simulink library "CAU_NXP_Car_Lib"  (R2016a)
settings: Solver=ode45  StartTime=0.0  StopTime=10.0  RelTol=1e-3
undefined symbols (not defined in the file or in its folder): s
settings Model: Creator=tfuser  LastModifiedBy=tfuser
settings DataIOCC: LimitDataPoints=on  SaveFormat=Array
settings DebuggingCC: AllowSymbolicDim=off
settings HardwareCC: ProdBitPerPointer=32  ProdLargestAtomicFloat=None  ProdIntDivRoundTo=Undefined  ProdEndianess=Unspecified  ProdWordSize=32  ProdHWDeviceType=32-bit Generic
settings ModelReferenceCC: PropagateSignalLabelsOutOfModel=off
settings ConfigComp: CovModelRefEnable=Off

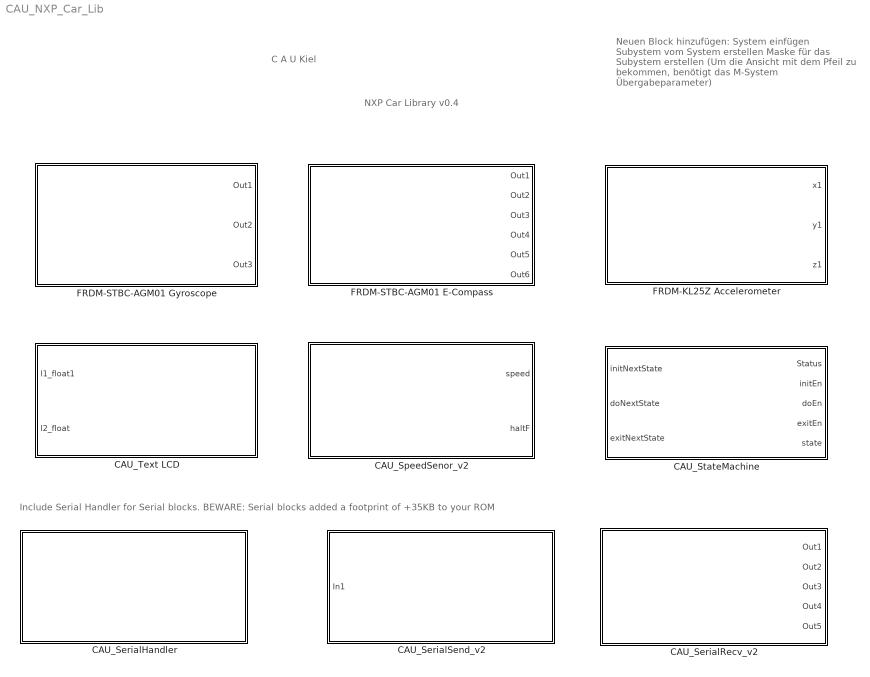
== system CAU_NXP_Car_Lib ==
  note: Include Serial Handler for Serial blocks. BEWARE: Serial blocks added a footprint of +35KB to your ROM
  note: Neuen Block hinzufügen:
      | System einfügen
      | Subystem vom System erstellen
      | Maske für das Subystem erstellen
      | (Um die Ansicht mit dem Pfeil zu bekommen,
      | benötigt das M-System Übergabeparameter)
  note: NXP Car Library v0.4
  note: C A U Kiel
  CAU_SerialHandler : Subsystem  mask{switchUART=0}
      mask prompts: switchUART "Switch UART (not implemented!)"
      mask help:
      | CAU_SerialHandler
      | Provides the pointer management to avoid two instances of mbeds serial object.
      mask TypeOptions switchUART: MATLAB System/switchUART
      mask Display:
      | pic = imread('resources/CAU_SerialHandler.png');
      | image(pic);
  CAU_SerialRecv_v2 : Subsystem  mask{quantToRecv=2, fullDigits=3, deciDigits=2, SampleTime=0.1}
      mask prompts: quantToRecv "Quantity of expected floating point numbers:"; fullDigits "Full Digits:"; deciDigits "Fractional digits:"; SampleTime "Simulink:blkprm_prompts:AllSrcBlksSampleTime"
      mask help:
      | Recieves serial data over UART/BT interface. The expected quantity parameter is crucial to match the incomming number of floats to act non-blocking! Output size is hard coded to 5* and output will be zero if there are less incomming numbers.
      |
      | Expected message format (ASCII coding): >+XXX.xx -YYY.yy ...
      | (Start char: ">", Seperator: Whitespace)
      |
      | * this output size is hard coded as constant property, as dealing with dynamic output length is not well supported by Simulink Coder.
      mask TypeOptions quantToRecv: MATLAB System/quantToRecv
      mask TypeOptions fullDigits: MATLAB System/fullDigits
      mask TypeOptions deciDigits: MATLAB System/deciDigits
      mask TypeOptions SampleTime: Constant1/SampleTime
      mask Display:
      | pic = imread('resources/SLBlock_Serial_Recv.png');
      | image(pic);
      | 
      | port_label('output',1,'f1');
      | port_label('output',2,'f2');
      | port_label('output',3,'f3');
      | port_label('output',4,'f4');
      | port_label('output',5,'f5');
  CAU_SerialSend_v2 : Subsystem  mask{quantToTrnf=2}
      mask prompts: quantToTrnf "Quantity to transfer:"
      mask help:
      | Sends a vector of floating points via UART/Bluetooth.
      | Numbers are formated to "+XXX.xx" with no range limitations (E-Notation is used)
      | Include State Machine!
      mask TypeOptions quantToTrnf: MATLAB System/quantToTrnf
      mask Display:
      | pic = imread('resources/SLBlock_Serial_Send.png');
      | image(pic);
      | 
      | port_label('input',1,'numVec');
  CAU_SpeedSenor_v2 : Subsystem  mask{WhichSensor=Left, SgmntWdth=36, ElpsdTMax=400, ChrTPT1=1/5, SampleTime=0.01}
      mask prompts: WhichSensor "Select Sensor:"; SgmntWdth "Segement width between two magnets in mm:"; ElpsdTMax "Maximum elapsed time in ms before stillstand detection, [300, 800]:"; ChrTPT1 "PT1 low pass: characteristic factor in respect to the block sample time [0, 10]:"; SampleTime "Simulink:blkprm_prompts:AllSrcBlksSampleTime"
      mask help: Measure car speed with magnets mounted inside the wheel.
      mask TypeOptions WhichSensor: MATLAB System/WhichSensor
      mask TypeOptions SgmntWdth: MATLAB System/SgmntWdth
      mask TypeOptions ElpsdTMax: MATLAB System/ElpsdTMax
      mask TypeOptions ChrTPT1: MATLAB System/ChrTPT1
      mask TypeOptions SampleTime: Constant1/SampleTime
      mask Display:
      | pic = imread('resources/speedsensor.png');
      | image(pic);
      | 
      | port_label('output',1,'speed');
      | port_label('output',2,'haltFlag');
  CAU_StateMachine : Subsystem  mask{SampleTime=0.1}
      mask prompts: SampleTime "Simulink:blkprm_prompts:AllSrcBlksSampleTime"
      mask TypeOptions SampleTime: Constant1/SampleTime
      mask Display:
      | pic = imread('resources/CAU_StateMachine.png');
      | image(pic);
      | 
      | port_label('output',1,'status');
      | port_label('output',2,'initEn');
      | port_label('output',3,'doEn');
      | port_label('output',4,'exitEn');
      | 
      | port_label('output',5,'state');
      | 
      | port_label('input',1,'initNext');
      | port_label('input',2,'doNext');
      | port_label('input',3,'exitNext');
  CAU_Text LCD : Subsystem  mask(Text LCD Display){}
      mask help:
      | TextLCD: print two floating numbers to the two lines of a HD44780 display
      |
      | IMPORTANT: add "-u_printf_float -u_scanf_float" to your <Linker> and <C++ Linker> options.
      |
      | Connected PINs : {PTC0}RS, {PTC7}E, {PTB8,PTB9,PTB10,PTB11}Data.
      | (TODO: To reduce the cables to two use a I2C implementation)
      mask Display:
      | pic = imread('resources/lcd.png');
      | image(pic);
      | 
      | port_label('input',1,'line1');
      | port_label('input',2,'line2');
  FRDM-KL25Z Accelerometer : Subsystem  SystemSampleTime=SystemSampleTime  mask(Accelerometer){WhichScale=+-2G, SystemSampleTime=-1, SampleTime=0.1}
      mask prompts: WhichScale "Full Scale:"; SystemSampleTime "Simulink:blkprm_prompts:AllBlksSampleTime"; SampleTime "Simulink:blkprm_prompts:AllSrcBlksSampleTime"
      mask help:
      | This Block reads out the data from the Accelerometer that is on the FRDM-KL25Z.
      |
      | Outputs 1-3 are the acceleration in x, y and z axis in m/(s^2).
      mask TypeOptions WhichScale: MATLAB System/WhichScale
      mask TypeOptions SystemSampleTime: SystemSampleTime
      mask TypeOptions SampleTime: CONST_g/SampleTime
      mask Display:
      | pic = imread('resources/acc_int.png');
      | image(pic);
      | 
      | port_label('output',1,'accel_x');
      | port_label('output',2,'accel_y');
      | port_label('output',3,'accel_z');
  FRDM-STBC-AGM01 E-Compass : Subsystem  SystemSampleTime=SystemSampleTime  mask(Accelerometer and Magnetometer){WhichScale=+-2G, SystemSampleTime=-1, SampleTime=0.1}
      mask prompts: WhichScale "Acc Full Scale:"; SystemSampleTime "Simulink:blkprm_prompts:AllBlksSampleTime"; SampleTime "Simulink:blkprm_prompts:AllSrcBlksSampleTime"
      mask help:
      | This Block reads out the data from the FXOS8700C 6-axis integrated e-compass that is on the FRDM-STBC-AGM01 Sensor Fusion Board.
      |
      | It reads out the values of the Accelerometer and the Magnetometer.
      | Outputs 1-3 are the acceleration in x, y and z axis in m/(s^2).
      | Outputs 4-6 are the magnetudes in x, y and z axis in uT.
      mask TypeOptions WhichScale: MATLAB System1/WhichScale
      mask TypeOptions SystemSampleTime: SystemSampleTime
      mask TypeOptions SampleTime: Constant1/SampleTime
      mask Display:
      | pic = imread('resources/acc_mag.png');
      | image(pic);
      | 
      | port_label('output',1,'accel_x');
      | port_label('output',2,'accel_y');
      | port_label('output',3,'accel_z');
      | port_label('output',4,'mag_x');
      | port_label('output',5,'mag_y');
      | port_label('output',6,'mag_z');
  FRDM-STBC-AGM01 Gyroscope : Subsystem  SystemSampleTime=SystemSampleTime  mask(Gyroscope){WhichScale=+-500rad/s, SystemSampleTime=-1, SampleTime=0.1}
      mask prompts: WhichScale "Full Scale:"; SystemSampleTime "Simulink:blkprm_prompts:AllBlksSampleTime"; SampleTime "Simulink:blkprm_prompts:AllSrcBlksSampleTime"
      mask help:
      | This Block reads out the data from the FXAS21002C 3-axis Gyroscope that is on the FRDM-STBC-AGM01 Sensor Fusion Board.
      |
      | It reads out the values of the Gyroscope.
      | Outputs 1-3 are the gyro-data in x, y and z axis in rad/s.
      mask TypeOptions WhichScale: MATLAB System/WhichScale
      mask TypeOptions SystemSampleTime: SystemSampleTime
      mask TypeOptions SampleTime: Constant1/SampleTime
      mask Display:
      | pic = imread('resources/gyro.png');
      | image(pic);
      | 
      | port_label('output',1,'gyro_x');
      | port_label('output',2,'gyro_y');
      | port_label('output',3,'gyro_z');

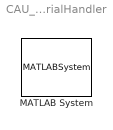
== system CAU_NXP_Car_Lib/CAU_SerialHandler ==
  MATLAB System : MATLABSystem  System=CAU_SerialHandler  switchUART=switchUART  SimulateUsing=Code generation
      mask Type: CAU_SerialHandler
      mask Display: disp('CAU_SerialHandler');

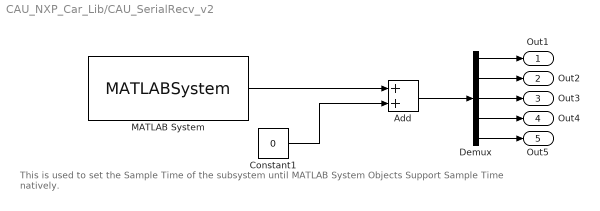
== system CAU_NXP_Car_Lib/CAU_SerialRecv_v2 ==
  note: This is used to set the Sample Time of the subsystem until MATLAB System Objects Support Sample Time natively.
  Add : Sum  AccumDataTypeStr=single
  Constant1 : Constant  Value=0  OutDataTypeStr=single  SampleTime=SampleTime
  Demux : Demux  Outputs=5
  MATLAB System : MATLABSystem  System=CAU_SerialRecv  quantToRecv=quantToRecv  fullDigits=fullDigits  deciDigits=deciDigits  SimulateUsing=Code generation
      mask Type: CAU_SerialRecv
      mask Display:
      | disp('CAU_SerialRecv');
      | port_label('output',1,'res');
  Out1 : Outport
  Out2 : Outport  Port=2
  Out3 : Outport  Port=3
  Out4 : Outport  Port=4
  Out5 : Outport  Port=5
  wires:
  Constant1/1 -> Add/2
  MATLAB System/1 -> Add/1
  Add/1 -> Demux/1
  Demux/1 -> Out1/1
  Demux/2 -> Out2/1
  Demux/3 -> Out3/1
  Demux/4 -> Out4/1
  Demux/5 -> Out5/1

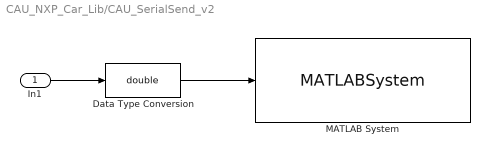
== system CAU_NXP_Car_Lib/CAU_SerialSend_v2 ==
  In1 : Inport
  Data Type Conversion : DataTypeConversion  OutDataTypeStr=double
  MATLAB System : MATLABSystem  System=CAU_SerialSend  quantToTrnf=quantToTrnf  SimulateUsing=Code generation
      mask Type: CAU_SerialSend
      mask Display:
      | disp('CAU_SerialSend');
      | port_label('input',1,'numVec');
  wires:
  In1/1 -> Data Type Conversion/1
  Data Type Conversion/1 -> MATLAB System/1

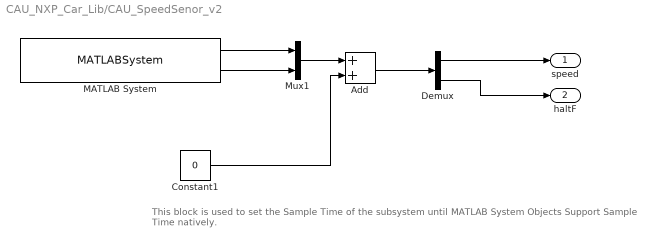
== system CAU_NXP_Car_Lib/CAU_SpeedSenor_v2 ==
  note: This block is used to set the Sample Time of the subsystem until MATLAB System Objects Support Sample Time natively.
  Add : Sum  AccumDataTypeStr=single
  Constant1 : Constant  Value=0  OutDataTypeStr=single  SampleTime=SampleTime
  Demux : Demux  Outputs=2
  MATLAB System : MATLABSystem  System=CAU_SpeedSensor  SgmntWdth=SgmntWdth  ElpsdTMax=ElpsdTMax  ChrTPT1=ChrTPT1  WhichSensor=Left  SimulateUsing=Code generation
      mask Type: CAU_SpeedSensor
      mask Display:
      | disp('CAU_SpeedSensor');
      | port_label('output',1,'speed');
      | port_label('output',2,'stillstand');
  Mux1 : Mux  Inputs=2
  speed : Outport
  haltF : Outport  Port=2
  wires:
  Constant1/1 -> Add/2
  Mux1/1 -> Add/1
  MATLAB System/2 -> Mux1/2
  Add/1 -> Demux/1
  Demux/2 -> haltF/1
  MATLAB System/1 -> Mux1/1
  Demux/1 -> speed/1

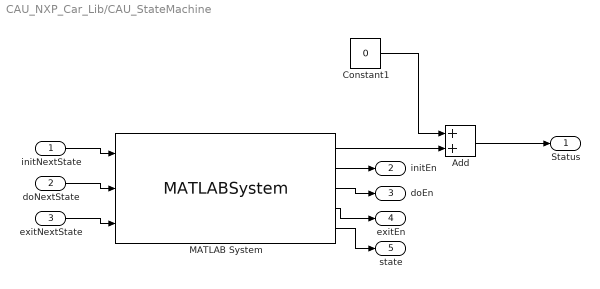
== system CAU_NXP_Car_Lib/CAU_StateMachine ==
  initNextState : Inport
  doNextState : Inport  Port=2
  exitNextState : Inport  Port=3
  Add : Sum  AccumDataTypeStr=single
  Constant1 : Constant  Value=0  OutDataTypeStr=single  SampleTime=SampleTime
  MATLAB System : MATLABSystem  System=CAU_StateMachine  SimulateUsing=Code generation
      mask Type: CAU_StateMachine
      mask Display:
      | disp('CAU_StateMachine');
      | port_label('input',1,'initNext');
      | port_label('input',2,'doNext');
      | port_label('input',3,'exitNext');
      | port_label('output',1,'status');
      | port_label('output',2,'initEn');
      | port_label('output',3,'doEn');
      | port_label('output',4,'exitEn');
      | port_label('output',5,'currState');
  Status : Outport
  initEn : Outport  Port=2
  doEn : Outport  Port=3
  exitEn : Outport  Port=4
  state : Outport  Port=5
  wires:
  Constant1/1 -> Add/1
  Add/1 -> Status/1
  initNextState/1 -> MATLAB System/1
  exitNextState/1 -> MATLAB System/3
  doNextState/1 -> MATLAB System/2
  MATLAB System/1 -> Add/2
  MATLAB System/4 -> exitEn/1
  MATLAB System/3 -> doEn/1
  MATLAB System/2 -> initEn/1
  MATLAB System/5 -> state/1

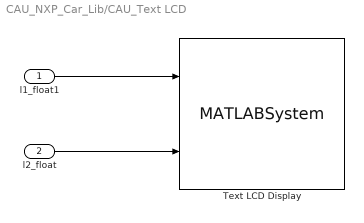
== system CAU_NXP_Car_Lib/CAU_Text LCD ==
  l1_float1 : Inport
  l2_float : Inport  Port=2
  Text LCD Display : MATLABSystem  System=TextLCD  SimulateUsing=Code generation
      mask Type: TextLCD
      mask Display:
      | disp('TextLCD');
      | port_label('input',1,'line1');
      | port_label('input',2,'line2');
  wires:
  l1_float1/1 -> Text LCD Display/1
  l2_float/1 -> Text LCD Display/2

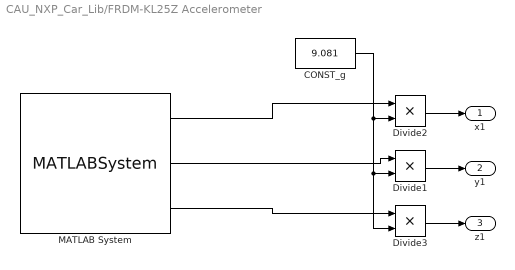
== system CAU_NXP_Car_Lib/FRDM-KL25Z Accelerometer ==
  CONST_g : Constant  Value=9.081  SampleTime=SampleTime
  Divide1 : Product  Inputs=**
  Divide2 : Product  Inputs=**
  Divide3 : Product  Inputs=**
  MATLAB System : MATLABSystem  System=MMA8451Q  WhichScale=+-2G  SimulateUsing=Code generation
      mask Type: MMA8451Q
      mask Display:
      | disp('MMA8451Q');
      | port_label('output',1,'accel_x');
      | port_label('output',2,'accel_y');
      | port_label('output',3,'accel_z');
  x1 : Outport
  y1 : Outport  Port=2
  z1 : Outport  Port=3
  wires:
  MATLAB System/3 -> Divide3/1
  CONST_g/1 -> Divide3/2, Divide1/2, Divide2/2
  MATLAB System/2 -> Divide1/1
  MATLAB System/1 -> Divide2/1
  Divide2/1 -> x1/1
  Divide1/1 -> y1/1
  Divide3/1 -> z1/1

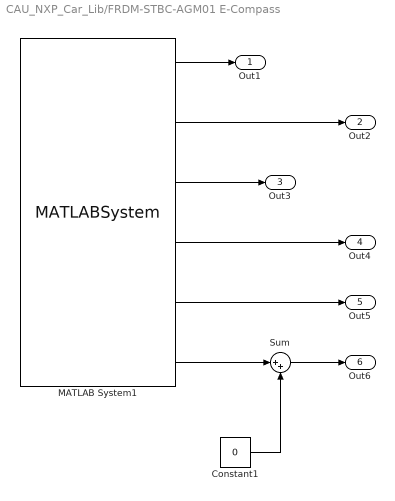
== system CAU_NXP_Car_Lib/FRDM-STBC-AGM01 E-Compass ==
  Constant1 : Constant  Value=0  OutDataTypeStr=single  SampleTime=SampleTime
  MATLAB System1 : MATLABSystem  System=FXOS8700C  WhichScale=+-2G  SimulateUsing=Code generation
      mask Type: FXOS8700C
      mask Display:
      | disp('FXOS8700C');
      | port_label('output',1,'accel_x');
      | port_label('output',2,'accel_y');
      | port_label('output',3,'accel_z');
      | port_label('output',4,'mag_x');
      | port_label('output',5,'mag_y');
      | port_label('output',6,'mag_z');
  Sum : Sum  Inputs=|++
  Out1 : Outport
  Out2 : Outport  Port=2
  Out3 : Outport  Port=3
  Out4 : Outport  Port=4
  Out5 : Outport  Port=5
  Out6 : Outport  Port=6
  wires:
  MATLAB System1/4 -> Out4/1
  MATLAB System1/2 -> Out2/1
  MATLAB System1/3 -> Out3/1
  MATLAB System1/5 -> Out5/1
  MATLAB System1/1 -> Out1/1
  Sum/1 -> Out6/1
  MATLAB System1/6 -> Sum/1
  Constant1/1 -> Sum/2

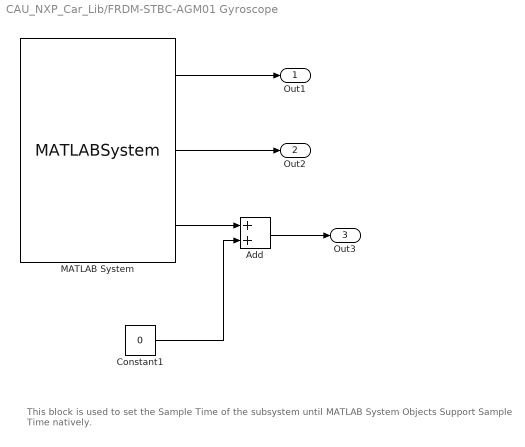
== system CAU_NXP_Car_Lib/FRDM-STBC-AGM01 Gyroscope ==
  note: This block is used to set the Sample Time of the subsystem until MATLAB System Objects Support Sample Time natively.
  Add : Sum  AccumDataTypeStr=single
  Constant1 : Constant  Value=0  OutDataTypeStr=single  SampleTime=SampleTime
  MATLAB System : MATLABSystem  System=FXAS21002C  WhichScale=+-500rad/s  SimulateUsing=Code generation
      mask Type: FXAS21002C
      mask Display:
      | disp('FXAS21002C');
      | port_label('output',1,'gyro_x');
      | port_label('output',2,'gyro_y');
      | port_label('output',3,'gyro_z');
  Out1 : Outport
  Out2 : Outport  Port=2
  Out3 : Outport  Port=3
  wires:
  MATLAB System/1 -> Out1/1
  MATLAB System/2 -> Out2/1
  Add/1 -> Out3/1
  MATLAB System/3 -> Add/1
  Constant1/1 -> Add/2
